simulink model "a2e2a"  (R2020a)
settings: Solver=VariableStepAuto  StartTime=0.0  StopTime=40000  RelTol=1e-3
libraries: eeGeneralControl x1
settings Model: EnablePacing=on  PacingRate=2  Creator=mumun  LastModifiedBy=mumun

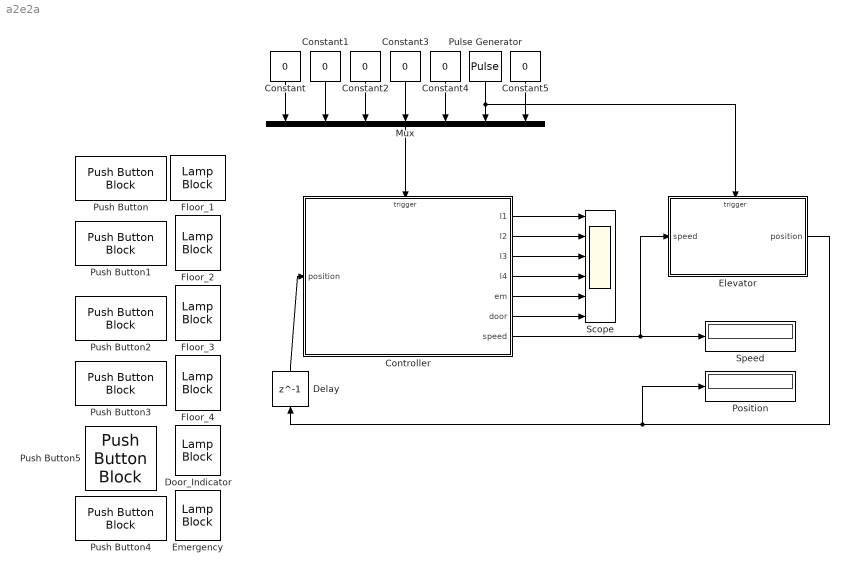
== system a2e2a ==
  Constant{,1..5} (6 alike) : Constant  Value=0
  Controller : Stateflow chart  TreatAsAtomicUnit=on
  Delay : Delay  DelayLength=1  DelayLengthUpperLimit=2  InputProcessing=Columns as channels (frame based)  SampleTime=1
  Door_Indicator : LampBlock  LabelPosition=Hide
  Elevator : Stateflow chart  TreatAsAtomicUnit=on
  Emergency : LampBlock  LabelPosition=Hide
  Floor_{1..4} (4 alike) : LampBlock  LabelPosition=Hide
  Mux : Mux  Inputs=7
  Position : Display
  Pulse Generator : DiscretePulseGenerator  PulseType=Time based  Period=1  PulseWidth=99
  Push Button : PushButtonBlock  ButtonText=Floor_1
  Push Button1 : PushButtonBlock  ButtonText=Floor_2
  Push Button2 : PushButtonBlock  ButtonText=Floor_3
  Push Button3 : PushButtonBlock  ButtonText=Floor_4
  Push Button4 : PushButtonBlock  ButtonText=Emergency
  Push Button5 : PushButtonBlock  ButtonText=Reset
  Scope : Scope  NumInputPorts=6
  Speed : Display
  wires:
  Constant/1 -> Mux/1
  Constant1/1 -> Mux/2
  Constant2/1 -> Mux/3
  Constant3/1 -> Mux/4
  Constant4/1 -> Mux/5
  Pulse Generator/1 -> Elevator/Trigger, Mux/6
  Mux/1 -> Controller/Trigger
  Constant5/1 -> Mux/7
  Controller/5(em) -> Scope/5
  Controller/6(door) -> Scope/6
  Elevator/1(position) -> Position/1, Delay/1
  Controller/7(speed) -> Elevator/1(speed), Speed/1
  Delay/1 -> Controller/1(position)
  Controller/1(l1) -> Scope/1
  Controller/2(l2) -> Scope/2
  Controller/3(l3) -> Scope/3
  Controller/4(l4) -> Scope/4

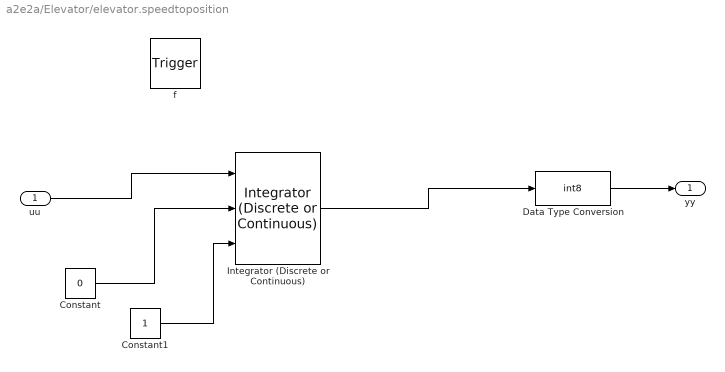
== system a2e2a/Elevator/elevator.speedtoposition ==
  uu : Inport  OutDataTypeStr=double  PortDimensions=1
  f : TriggerPort  TriggerType=function-call  VariantControl=(inherit)
      settings: CopyFcn=Stateflow.SLINSF.SimulinkMan.removeBlockPreDeleteFcn  PreDeleteFcn=Stateflow.SLINSF.SimulinkMan.unsafePredeleteFcn
  Constant : Constant  Value=0
  Constant1 : Constant
  Data Type Conversion : DataTypeConversion  OutDataTypeStr=int8  RndMeth=Round
  Integrator (Discrete or Continuous) : eeGeneralControl/Integrator (Discrete or Continuous)  LabelModeActiveChoice=Discrete  ExternalReset=level  LimitType=Anti-windup  B=4  A=0  Ts=-1
      settings: SourceProductBaseCode=PS
  yy : Outport
  wires:
  uu/1 -> Integrator (Discrete or Continuous)/1
  Integrator (Discrete or Continuous)/1 -> Data Type Conversion/1
  Data Type Conversion/1 -> yy/1
  Constant/1 -> Integrator (Discrete or Continuous)/2
  Constant1/1 -> Integrator (Discrete or Continuous)/3

== stateflow chart a2e2a/Elevator ==
  state elevator
    en, du: position=speedtoposition(speed)
    state yy = speedtoposition(uu) [function]
  (default) -> elevator
  data: uu function_input double size=1; yy function_output; speed input; position output
  events: pulse input EITHER_EDGE_EVENT

== stateflow chart a2e2a/Controller ==
  settings: executeAtInitialization=1
  state controller
    en: em=0; go1=0; go2=0; go3=0; go4=0; door=0;reached=0;t=0; l1=0;l2=0;l3=0;l4=0;
    on Floor_1:  go1=1;l1=1;
    on Floor_2:  go2=1;l2=1;
    on Floor_3:  go3=1;l3=1;
    on Floor_4:  go4=1;l4=1;
    on emergency: em=1;
    on restart: em=0;
    en, du: controllerlogic();
    state floor3
      state closed
        du:door=0;
      state open
        en,du: door=1;l3=0;
        en,du: t=elapsed(sec);
        exit: door=0;go3=0;
      (default) -> controller.floor3.closed
      controller.floor3.open -> controller.floor3.closed : [t>=5]
      controller.floor3.closed -> controller.floor3.open : [l3==1]
    state floor2
      state closed
        du:door=0;
      state open
        en,du: door=1;l2=0;
        en,du: t=elapsed(sec);
        exit: door=0;go2=0;
      (default) -> controller.floor2.closed
      controller.floor2.open -> controller.floor2.closed : [t>=5]
      controller.floor2.closed -> controller.floor2.open : [l2==1]
    state floor4
      state closed
        du:door=0;
      state open
        en,du: door=1;l4=0;
        en,du: t=elapsed(sec);
        exit: door=0;go4=0;
      (default) -> controller.floor4.closed
      controller.floor4.open -> controller.floor4.closed : [t>=5]
      controller.floor4.closed -> controller.floor4.open : [l4==1]
    state floor1
      state closed
        du:door=0;
      state open
        en,du: door=1;l1=0;
        en,du: t=elapsed(sec);
        exit: door=0;go1=0;
      (default) -> controller.floor1.closed
      controller.floor1.open -> controller.floor1.closed : [t>=5]
      controller.floor1.closed -> controller.floor1.open : [l1==1]
    floor3 -> floor2 [order 2] : [position==2]
    floor2 -> floor3 [order 1] : [position==3]
    floor2 -> floor1 [order 2] : [position==1]
    floor1 -> floor2 : [position==2]
    floor4 -> floor3 : [position==3]
    floor3 -> floor4 [order 1] : [position==4]
    (default) -> floor1
  (default) -> controller
  data: l1 output double size=1; l2 output double size=1; l3 output double size=1; l4 output double size=1; em output double size=1; door output double size=1; speed output double size=1; position input double size=1; reached local double size=1; t local double size=1; go1 local double size=1; go2 local double size=1; go3 local double size=1; go4 local double size=1
  events: Floor_1 input RISING_EDGE_EVENT; Floor_2 input RISING_EDGE_EVENT; Floor_3 input RISING_EDGE_EVENT; Floor_4 input RISING_EDGE_EVENT; emergency input RISING_EDGE_EVENT; pulse input EITHER_EDGE_EVENT; restart input RISING_EDGE_EVENT
  function controllerlogic:
    | function controllerlogic
    | max_speed= 0.2;
    | current_floor= round(position);
    | % destination_floor= 1;
    | % go=1;
    | 
    | if em == 0 && go1==1
    |     destination_floor= 1;
    |         if destination_floor-current_floor==0
    |             speed= 0;
    |             go1=0;
    |         elseif destination_floor-current_floor> 0
    |             speed= max_speed;          
    |         elseif destination_floor-(current_floor+1)< 0
    |             speed= -1*max_speed;
    |         end       
    | elseif em == 0 && go2==1
    |     destination_floor= 2;
    |         if destination_floor-current_floor==0
    |             speed= 0;
    |             go2=0;
    |         elseif destination_floor-current_floor> 0
    |             speed= max_speed;          
    |         elseif destination_floor-(current_floor+1)< 0
    |             speed= -1*max_speed;
    |         end
    | elseif em == 0 && go3==1
    |     destination_floor= 3;
    |         if destination_floor-current_floor==0
    |             speed= 0;
    |             go3=0;
    |         elseif destination_floor-current_floor> 0
    |             speed= max_speed;          
    |         elseif destination_floor-(current_floor+1)< 0
    |             speed= -1*max_speed;
    |         end
    | elseif em == 0 && go4==1
    |     destination_floor= 4;
    |         if destination_floor-current_floor==0
    |             speed= 0;
    |             go4=0;
    |         elseif destination_floor-current_floor> 0
    |             speed= max_speed;          
    |         elseif destination_floor-(current_floor+1)< 0
    |             speed= -1*max_speed;
    |         end        
    | elseif em == 1
    |     destination_floor= 1;
    |         if destination_floor-current_floor==0
    |             speed= 0;
    |             go2=0;
    |             go3=0;
    |             go4=0;
    |             l2=0;
    |             l3=0;
    |             l4=0;
    |         elseif destination_floor-current_floor> 0
    |             speed= max_speed;
    |         elseif destination_floor-(current_floor+1)< 0
    |             speed= -1*max_speed;
    |         end
    | end
    | end
